simulink subsystem "dsmFun"  (R2021b)
settings: Solver=VariableStepAuto  StartTime=0.0  StopTime=10.0  RelTol=1e-3
undefined symbols (not defined in the file): dMin, dScale, dsmConst, Length
libraries: fl_lib x2, nesl_utility x2
settings Model: Creator=Jiaqi  LastModifiedBy=silen

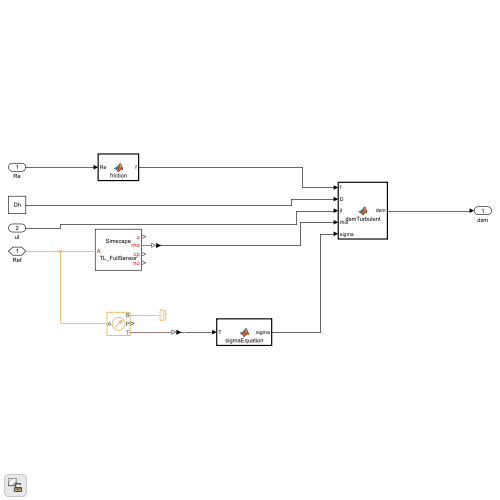
[thumbnail: Simulink's stored preview of the top-level diagram]
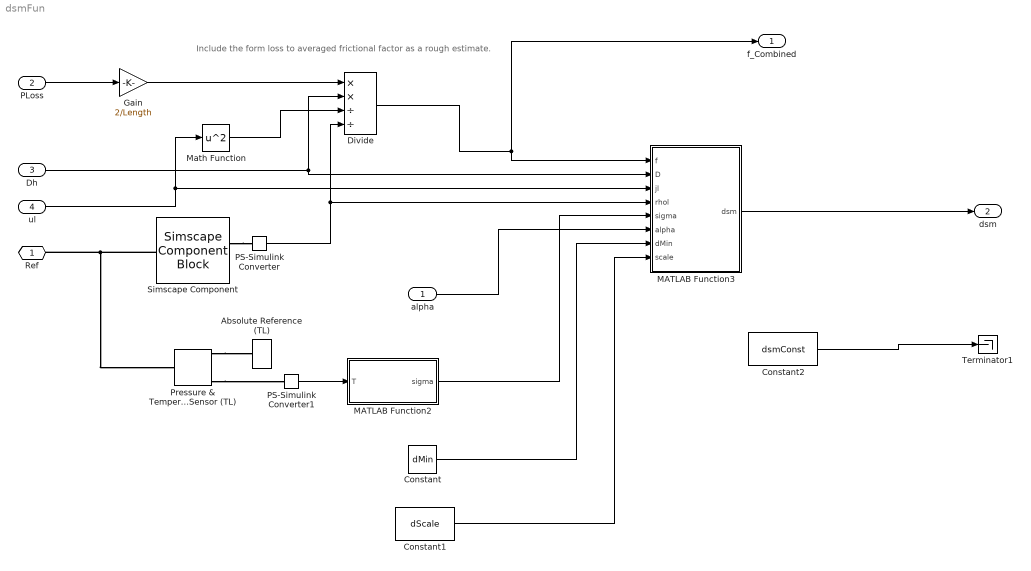
== system dsmFun ==
  note: Include the form loss to averaged frictional factor as a rough estimate.
  alpha : Inport
  PLoss : Inport  Port=2
  Dh : Inport  Port=3
  ul : Inport  Port=4
  Absolute Reference (TL) : fl_lib/Thermal Liquid/Elements/Absolute Reference (TL)
      settings: SourceProductBaseCode=SS
  Constant : Constant  Value=dMin
  Constant1 : Constant  Value=dScale
  Constant2 : Constant  Value=dsmConst
  Divide : Product  Inputs=**//
  Gain : Gain  Gain=2/Length
  MATLAB Function2 : MATLAB Function  TreatAsAtomicUnit=on
  MATLAB Function3 : MATLAB Function  TreatAsAtomicUnit=on
  Math Function : Math  Operator=square  SaturateOnIntegerOverflow=on
  PS-Simulink Converter : nesl_utility/PS-Simulink Converter  PhysicalDomain=network_engine_domain  SubClassName=ps_output  LeftPortType=input  RightPortType=output  PseudoPeriodic=off  Frequencies=[]  Unit=inherit  AffineConversion=off
      settings: SourceProductBaseCode=PW,SS
  PS-Simulink Converter1 : nesl_utility/PS-Simulink Converter  PhysicalDomain=network_engine_domain  SubClassName=ps_output  LeftPortType=input  RightPortType=output  PseudoPeriodic=off  Frequencies=[]  Unit=inherit  AffineConversion=off
      settings: SourceProductBaseCode=PW,SS
  Pressure & Temperature Sensor (TL) : fl_lib/Thermal Liquid/Sensors/Pressure & Temperature Sensor (TL)
      settings: SourceProductBaseCode=SS  InternalSimscapePortConfiguration="{\"Bottom\":[],\"Left\":[{\"id\":\"A\",\"label\":\"A\",\"type\":\"foundation.thermal_liquid.thermal_liquid\"}],\"Right\":[{\"id\":\"B\",\"label\":\"B\",\"type\":\"foundation.thermal_liquid.thermal_liquid\"},{\"id\":\"P\",\"label\":\"P\",\"type\":\"output\"},{\"id\":\"T\",\"label\":\"T\",\"type\":\"output\"}],\"Top\":[]}"
  Simscape Component : SimscapeComponentBlock  SourceFile=TL_FullSensor  ComponentPath=TL_FullSensor  ComponentVariants="[\"TL_FullSensor\"]"  ComponentVariantNames="[\"TL_FullSensor\"]"  ClassName=TL_FullSensor  SchemaVersion=1
      settings: CopyFcn=simscape.engine.sli.internal.componentblockcallback(gcbh,'COPY')  PreCopyFcn=simscape.engine.sli.internal.componentblockcallback(gcbh,'PRECOPY')  PreDeleteFcn=simscape.engine.sli.internal.componentblockcallback(gcbh,'PREDELETE')  InternalSimscapePortConfiguration="{\"Bottom\":[],\"Left\":[{\"id\":\"A\",\"label\":\"A\",\"type\":\"foundation.thermal_liquid.thermal_liquid\"}],\"Right\":[{\"id\":\"U\",\"label\":\"u\",\"type\":\"output\"},{\"id\":\"RHO\",\"label\":\"rho\",\"type\":\"output\"},{\"id\":\"CP\",\"label\":\"cp\",\"type\":\"output\"},{\"id\":\"NU\",\"label\":\"nu\",\"type\":\"output\"}],\"Top\":[]}"
      mask Type: Thermodynamic Properties Sensor (TL)
  Terminator1 : Terminator
  Ref : PMIOPort  Side=Right
  f_Combined : Outport
  dsm : Outport  Port=2
  wires:
  PS-Simulink Converter/1 -> MATLAB Function3/4(rhol), Divide/4
  ul/1 -> MATLAB Function3/3(jl), Math Function/1
  PS-Simulink Converter1/1 -> MATLAB Function2/1(T)
  MATLAB Function2/1(sigma) -> MATLAB Function3/5(sigma)
  Dh/1 -> Divide/2, MATLAB Function3/2(D)
  PLoss/1 -> Gain/1
  Gain/1 -> Divide/1
  Math Function/1 -> Divide/3
  Divide/1 -> f_Combined/1, MATLAB Function3/1(f)
  alpha/1 -> MATLAB Function3/6(alpha)
  Constant/1 -> MATLAB Function3/7(dMin)
  Constant1/1 -> MATLAB Function3/8(scale)
  MATLAB Function3/1(dsm) -> dsm/1
  Constant2/1 -> Terminator1/1
  connections:
  Ref/RConn1 -- Pressure & Temperature Sensor (TL)/LConn1 -- Simscape Component/LConn1
  Pressure & Temperature Sensor (TL)/RConn1 -- Absolute Reference (TL)/LConn1
  Simscape Component/RConn2 -- PS-Simulink Converter/LConn1
  Pressure & Temperature Sensor (TL)/RConn3 -- PS-Simulink Converter1/LConn1

== matlab function dsmFun/MATLAB Function2 ==
  data: T input; sigma output
function sigma = sigmaEquation(T)

T = T-273.15;
sigma = (235.5-0.09*T)*0.001; %Source from solubility in FLiBe by WATSON et al.

end

== matlab function dsmFun/MATLAB Function3 ==
  settings: updateMethod=DISCRETE
  data: f input; D input; jl input; rhol input; sigma input; dsm output; alpha input; dMin input; scale input
function dsm = dsmTurbulent(f,D,jl,rhol,sigma,alpha,dMin,scale)

f = abs(f);
jl = abs(jl);
rhol = abs(rhol);
sigma = abs(sigma);
%alpha = abs(alpha);

dissipation = jl^3/2/D*f;
dsm = scale*0.725/(rhol/sigma)^0.6/dissipation^0.4;
dsm = max(dsm,dMin);
x = -atanh(2*dMin/dsm-1);
dsm = max(dsm*(0.5 + 0.5*tanh(alpha*100-x)),1e-5);
%dsm = min(dsm,dMin*(1+alpha.^2))
dsm = min(dsm,D);

end
